simulink model "Three_Phase_Half_Controlled_Rectifier_RLE_GENERATOR_Load"  (R2018a)
settings: Solver=VariableStepAuto  StartTime=0.0  StopTime=1  RelTol=1e-3
libraries: powerlib x17, powerlib_meascontrol x7
settings Model: Creator=ozie  LastModifiedBy=ozie

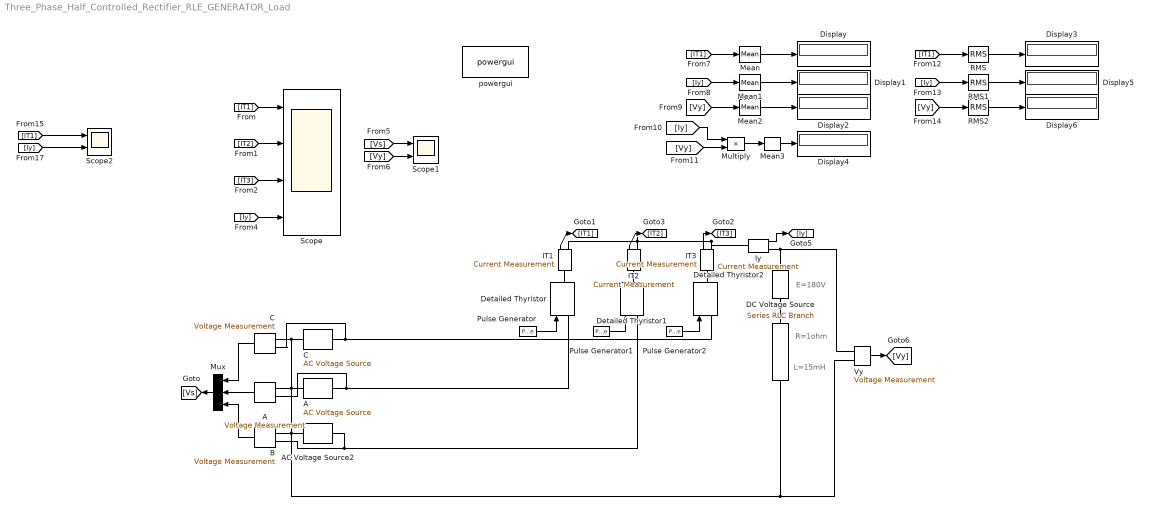
== system Three_Phase_Half_Controlled_Rectifier_RLE_GENERATOR_Load ==
  note: L=15mH
  note: E=180V
  note: R=1ohm
  "   " : powerlib/Elements/Series RLC Branch  LConnTagsString=__new0  RConnTagsString=__new0  BranchType=RL  Resistance=1  Inductance=15e-3  SetiL0=off  InitialCurrent=0  Capacitance=1e-6  Setx0=off  InitialVoltage=0  Measurements=None
  A : powerlib/Electrical Sources/AC Voltage Source  Amplitude=220*sqrt(2)  Phase=0  Frequency=50  SampleTime=0  Measurements=None  BusType=swing  Pref=10e3  Qref=0  Qmin=-inf  Qmax=+inf
  "A  " : powerlib/Measurements/Voltage Measurement  PhasorSimulation=off  OutputType=Complex  PSBequivalent=0
  AC Voltage Source2 : powerlib/Electrical Sources/AC Voltage Source  Amplitude=220*sqrt(2)  Phase=-120  Frequency=50  SampleTime=0  Measurements=None  BusType=swing  Pref=10e3  Qref=0  Qmin=-inf  Qmax=+inf
  "B  " : powerlib/Measurements/Voltage Measurement  PhasorSimulation=off  OutputType=Complex  PSBequivalent=0
  C : powerlib/Electrical Sources/AC Voltage Source  Amplitude=220*sqrt(2)  Phase=120  Frequency=50  SampleTime=0  Measurements=None  BusType=swing  Pref=10e3  Qref=0  Qmin=-inf  Qmax=+inf
  "C  " : powerlib/Measurements/Voltage Measurement  PhasorSimulation=off  OutputType=Complex  PSBequivalent=0
  DC Voltage Source : powerlib/Electrical Sources/DC Voltage Source  Amplitude=180  Measurements=None
  Detailed Thyristor : powerlib/Power Electronics/Detailed Thyristor  Ron=0.001  Lon=1e-3  Vf=0.0001  IL=0.1  Tq=100e-6  IC=0  Rs=500  Cs=250e-9  Measurements=off
      settings: SourceProductName=Simscape Power Systems  SourceProductBaseCode=PS
  Detailed Thyristor1 : powerlib/Power Electronics/Detailed Thyristor  Ron=0.001  Lon=1e-3  Vf=0.0001  IL=0.1  Tq=100e-6  IC=0  Rs=500  Cs=250e-9  Measurements=off
      settings: SourceProductName=Simscape Power Systems  SourceProductBaseCode=PS
  Detailed Thyristor2 : powerlib/Power Electronics/Detailed Thyristor  Ron=0.001  Lon=1e-3  Vf=0.0001  IL=0.1  Tq=100e-6  IC=0  Rs=500  Cs=250e-9  Measurements=off
      settings: SourceProductName=Simscape Power Systems  SourceProductBaseCode=PS
  Display{,1..6} (7 alike) : Display
      Display4 settings: Format=bank
  IT1 : powerlib/Measurements/Current Measurement  PhasorSimulation=off  OutputType=Complex  PSBequivalent=0
  IT2 : powerlib/Measurements/Current Measurement  PhasorSimulation=off  OutputType=Complex  PSBequivalent=0
  IT3 : powerlib/Measurements/Current Measurement  PhasorSimulation=off  OutputType=Complex  PSBequivalent=0
  Iy : powerlib/Measurements/Current Measurement  PhasorSimulation=off  OutputType=Complex  PSBequivalent=0
  Mean{,1..3} (4 alike) : powerlib_meascontrol/Measurements/Mean  Freq=50  Vinit=0  Ts=0
  Multiply : Product
  Mux : Mux  Inputs=3
  Pulse Generator : DiscretePulseGenerator  PulseType=Time based  Period=1/50  PulseWidth=5  PhaseDelay=0.01*(150/180)
  Pulse Generator1 : DiscretePulseGenerator  PulseType=Time based  Period=1/50  PulseWidth=5  PhaseDelay=0.01*(270/180)
  Pulse Generator2 : DiscretePulseGenerator  PulseType=Time based  Period=1/50  PulseWidth=5  PhaseDelay=0.01*(390/180)
  RMS : powerlib_meascontrol/Measurements/RMS  TrueRMS=on  Freq=60  RMSInit=120  Ts=0
  RMS1 : powerlib_meascontrol/Measurements/RMS  TrueRMS=on  Freq=60  RMSInit=120  Ts=0
  RMS2 : powerlib_meascontrol/Measurements/RMS  TrueRMS=on  Freq=60  RMSInit=120  Ts=0
  Scope : Scope  NumInputPorts=4
  Scope1 : Scope  NumInputPorts=2
  Scope2 : Scope  NumInputPorts=2
  Vy : powerlib/Measurements/Voltage Measurement  PhasorSimulation=off  OutputType=Complex  PSBequivalent=0
  powergui : powerlib/powergui  Priority=1  SimulationMode=Continuous  SampleTime=50e-6  frequency=60  Iterations=50  frequencyindice=50  Pbase=100e6  ErrMax=1e-4  UnitsV=kV  UnitsW=MW  buscounter=0  FunctionMessages=off  echomessages=off  EnableUseOfTLC=off  CurrentSourceSwitches=off  DisableSnubberDevices=off  DisableRonSwitches=off  DisableVfSwitches=off  DisplayEquations=off  SolverType=Tustin/Backward Euler (TBE)  Interpol=off  ExternalGateDelay=off  methode=off  Ts=100  x0status=blocks  SPID=on  SwTol=0  HookPort=off  RestoreLinks=warning  ResistiveCurrentMeasurement=off  Frange=[0:2:500]  Ylog=off  Xlog=on  ShowGrid=off  save=off  variable=ZData  structure=0  ZoomFFT=off  StartTime=0.0  cycles=1  DisplayStyle=1  fundamental=60  FreqAxis=off  MaxFrequency=1000  frequencyindicesteady=1  RmsSteady=1  display=off
  wires:
  [Vy] -> Multiply/2
  RMS1/1 -> Display5/1
  [Iy] -> RMS1/1
  [IT1] -> RMS/1
  [Vy] -> Mean2/1
  RMS2/1 -> Display6/1
  [Vy] -> RMS2/1
  RMS/1 -> Display3/1
  Mean/1 -> Display/1
  [Iy] -> Multiply/1
  Multiply/1 -> Mean3/1
  Iy/1 -> [Iy]
  Mux/1 -> [Vs]
  IT2/1 -> [IT2]
  Vy/1 -> [Vy]
  Mean3/1 -> Display4/1
  IT1/1 -> [IT1]
  "A  "/1 -> Mux/2
  "B  "/1 -> Mux/3
  IT3/1 -> [IT3]
  Mean1/1 -> Display1/1
  [IT1] -> Mean/1
  Mean2/1 -> Display2/1
  [Iy] -> Mean1/1
  [Iy] -> Scope/4
  "C  "/1 -> Mux/1
  Pulse Generator1/1 -> Detailed Thyristor1/1
  [Vs] -> Scope1/1
  [Vy] -> Scope1/2
  [IT3] -> Scope/3
  [IT1] -> Scope/1
  [IT2] -> Scope/2
  [Iy] -> Scope2/2
  Pulse Generator2/1 -> Detailed Thyristor2/1
  Pulse Generator/1 -> Detailed Thyristor/1
  [IT1] -> Scope2/1
  connections:
  Detailed Thyristor1/LConn1 -- AC Voltage Source2/RConn1 -- "B  "/LConn1
  "   "/RConn1 -- C/LConn1 -- "C  "/LConn2 -- "A  "/LConn2 -- A/LConn1 -- "B  "/LConn2 -- AC Voltage Source2/LConn1 -- Vy/LConn2
  IT2/RConn1 -- Iy/LConn1 -- IT3/RConn1 -- IT1/RConn1
  "A  "/LConn1 -- A/RConn1 -- Detailed Thyristor/LConn1
  "C  "/LConn1 -- C/RConn1 -- Detailed Thyristor2/LConn1
  Vy/LConn1 -- DC Voltage Source/LConn1 -- Iy/RConn1
  Detailed Thyristor2/RConn1 -- IT3/LConn1
  IT1/LConn1 -- Detailed Thyristor/RConn1
  IT2/LConn1 -- Detailed Thyristor1/RConn1
  DC Voltage Source/RConn1 -- "   "/LConn1
